simulink model "sgm_iox_io397_analog_loopback"  (R2018a)
settings: Solver=ode4  StartTime=0.0  StopTime=0.175  FixedStep=1/Fs  MaxStep=0.5  RelTol=1e-3  EnableMultiTasking=on
model workspace (MAT data in the model file):
  C = 1e-07
  Fs = 5000
  R = 18000
undefined symbols (not defined in the file): IO397
libraries: speedgoatlib_fpga_analog_io x2, speedgoatlib_fpga x1
Description:
  | This model demonstrates three different representations
  | of a 2nd-Order system.
settings Model: ModifiedHistory="05 Feb 2002  Created."  SimulationMode=external  ExtModeTrigMode=oneshot  ExtModeArmWhenConnect=off  Creator=Douglas G. Jones  LastModifiedBy=daniel.fonte
settings SolverCC: ConcurrentTasks=on  PositivePriorityOrder=on  AutoInsertRateTranBlk=on
settings DataIOCC: SaveFormat=StructureWithTime  SaveState=on
settings OptimizationCC: BlockReduction=off  BooleanDataType=off  OptimizeBlockIOStorage=off  BufferReuse=off  GlobalBufferReuse=off  ExpressionFolding=off  ExpressionDepthLimit=2147483647  LocalBlockOutputs=off  InitFltsAndDblsToZero=on  OptimizeDataStoreBuffers=off  BusAssignmentInplaceUpdate=off
settings DebuggingCC: SaveWithParameterizedLinksMsg=none  UnderspecifiedInitializationDetection=Classic  MergeDetectMultiDrivingBlocksExec=none  SignalResolutionControl=TryResolveAllWithWarning  FcnCallInpInsideContextMsg=warning  AllowSymbolicDim=off  StateNameClashWarn=warning  SFUnexpectedBacktrackingDiag=warning  SFNoUnconditionalDefaultTransitionDiag=warning  SFExecutionAtInitializationDiag=none
settings HardwareCC: ProdBitPerPointer=32  ProdBitPerSizeT=32  ProdBitPerPtrDiffT=32  ProdLargestAtomicFloat=None  ProdWordSize=32  ProdLongLongMode=on  ProdHWDeviceType=Generic->32-bit x86 compatible
settings ModelReferenceCC: PropagateSignalLabelsOutOfModel=off
settings RTWCC: SystemTargetFile=slrt.tlc  TemplateMakefile=slrt_default_tmf  Description=Simulink Real-Time  RTWVerbose=off  Toolchain=Simulink Real-Time Toolchain  BuildConfiguration=Faster Runs  CodeExecutionProfiling=on  RTWCompilerOptimization=on
settings CodeAppCC: StateflowObjectComments=on
settings SimulinkRealTimeCC: SupportVariableSizeSignals=on  RL32LogTETModifier=off  xPCConcurrentTasks=on
settings ConfigComp: CovMetricSettings=dw  CovSaveCumulativeToWorkspaceVar=on  CovSaveSingleToWorkspaceVar=on  CovExternalEMLEnable=off  CovSFcnEnable=off
settings SimscapeCC: SimscapeNormalizeSystem=off
settings ConfigurationSet: Description=SimMechanics 2G

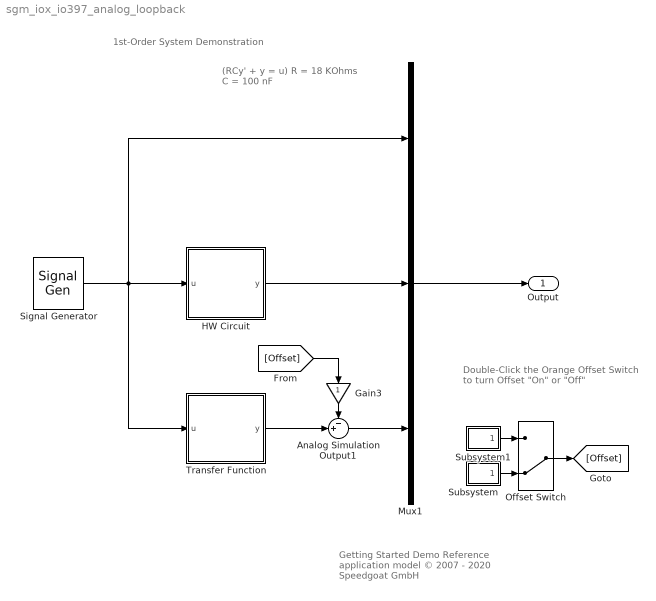
== system sgm_iox_io397_analog_loopback ==
  note: 1st-Order System Demonstration
  note: (RCy' + y = u)
      | R = 18 KOhms
      | C = 100 nF
  note: Double-Click
      | the Orange Offset Switch
      | to turn Offset "On" or "Off"
  note: Getting Started Demo
      | Reference application model
      | © 2007 - 2020 Speedgoat GmbH
  Analog Simulation Output1 : Sum  Inputs=-+|  SaturateOnIntegerOverflow=on  InputSameDT=on  OutDataTypeStr=Inherit: Same as first input
  Gain3 : Gain
  HW Circuit : Subsystem  TreatAsAtomicUnit=on
  Mux1 : Mux  Inputs=3
  Offset Switch : ManualSwitch  CurrentSetting=0
  Signal Generator : SignalGenerator  WaveForm=square  Amplitude=4  Frequency=10
  Subsystem : Subsystem
      mask Display: disp('Off')
  Subsystem1 : Subsystem
      mask Display: disp('On')
  Transfer Function : Subsystem
  Output : Outport
  wires:
  Signal Generator/1 -> HW Circuit/1(u), Transfer Function/1(u), Mux1/1
  Mux1/1 -> Output/1
  HW Circuit/1(y) -> Mux1/2
  Transfer Function/1(y) -> Analog Simulation Output1/2
  Gain3/1 -> Analog Simulation Output1/1
  Analog Simulation Output1/1 -> Mux1/3
  [Offset] -> Gain3/1
  Offset Switch/1 -> [Offset]
  Subsystem1/1(Out 1) -> Offset Switch/1
  Subsystem/1(Out 1) -> Offset Switch/2

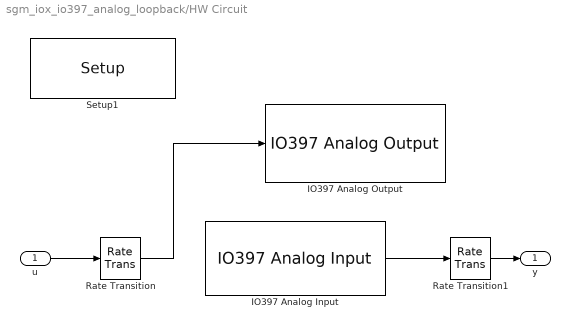
== system sgm_iox_io397_analog_loopback/HW Circuit ==
  u : Inport
  IO397 Analog Input : speedgoatlib_fpga_analog_io/IO397 Analog Input  id=1  chan=2  range=+-5 V  trigger=Initiator  ts=0.001  pciSlot=-1  board=IO397-50k
      settings: SourceProductName=Simulink Real-Time: Speedgoat I/O Driver Library
  IO397 Analog Output : speedgoatlib_fpga_analog_io/IO397 Analog Output  id=1  chan=1  initVal=0  resetVal=0  ts=0.001  pciSlot=-1  board=IO397-50k  span=+-5 V
      settings: SourceProductName=Simulink Real-Time: Speedgoat I/O Driver Library
  Rate Transition : RateTransition  Deterministic=off
  Rate Transition1 : RateTransition  Deterministic=off
  Setup1 : speedgoatlib_fpga/Setup/Setup  board=IO397-50k  id=1  device_id=1  frontIO=None  rearIO=None  bitstreamFile=speedgoat_IO397_50k_CI_IO397_DUT_DEMO  rev=1.0  timestamp_string=05/10/17 09:15:16  fpgaFreq=75 MHz  fpgaTick=13.33 ns  ProgSpiFlash=off  ProgBPIFlash=off  pciSlot=-1  PullRPort0=pull-up 3.3V  VioPort0=3.3V  PullRPort1=pull-up 3.3V  VioPort1=3.3V  PullRPort2=pull-up 3.3V  VioPort2=3.3V  PullRPort3=pull-up 3.3V  VioPort3=3.3V  PullRPort4=pull-up 3.3V  VioPort4=3.3V  PullRPort5=pull-up 3.3V  VioPort5=3.3V  PullRPort6=pull-up 3.3V  VioPort6=3.3V  PullRPort15=pull-up 3.3V  PullRPort31=pull-up 3.3V  PullRPort47=pull-up 3.3V  PullRPort63=pull-up 3.3V
      settings: SourceProductName=Simulink Real-Time: Speedgoat I/O Driver Library
  y : Outport
  wires:
  u/1 -> Rate Transition/1
  IO397 Analog Input/1 -> Rate Transition1/1
  Rate Transition/1 -> IO397 Analog Output/1
  Rate Transition1/1 -> y/1

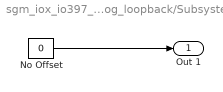
== system sgm_iox_io397_analog_loopback/Subsystem ==
  No Offset : Constant  Value=0
  Out 1 : Outport
  wires:
  No Offset/1 -> Out 1/1

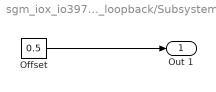
== system sgm_iox_io397_analog_loopback/Subsystem1 ==
  Offset : Constant  Value=0.5
  Out 1 : Outport
  wires:
  Offset/1 -> Out 1/1

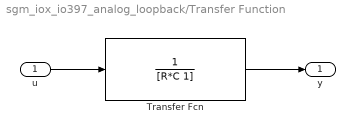
== system sgm_iox_io397_analog_loopback/Transfer Function ==
  u : Inport
  Transfer Fcn : TransferFcn  Denominator=[R*C 1]
  y : Outport
  wires:
  u/1 -> Transfer Fcn/1
  Transfer Fcn/1 -> y/1
